simulink model "FullDynamics_Model2"  (R2018b)
settings: Solver=FixedStepAuto  StartTime=0.0  StopTime=inf  FixedStep=0.01  RelTol=1e-3
undefined symbols (not defined in the file): aMode
libraries: robotlib x6, autolibshared x1, autolibsharedcommon x1
settings Model: Creator=ivory  LastModifiedBy=ivory

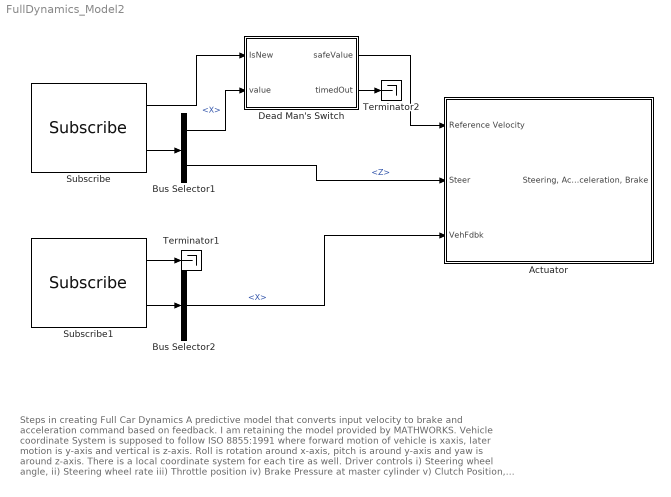
== system FullDynamics_Model2 ==
  note: Steps in creating Full Car Dynamics
      | A predictive model that converts input velocity
      | to brake and acceleration command based on feedback.
      | I am retaining the model provided by MATHWORKS.
      | Vehicle coordinate System is supposed to follow ISO
      | 8855:1991 where forward motion of vehicle is xaxis, later
      | motion is y-axis and vertical is z-axis. Roll is rotation around
      | x-axis, pitch is around y-axis and yaw is around z-axis. There
      | is a local coordinate system for each tire as well.
      | Driver controls i) Steering wheel angle, ii) Steering wheel rate
      | iii) Throttle position iv) Brake Pressure at master cylinder
      | v) Clutch Position, vi) Gear shift Position
      | Out of interests may be: i) Vehicle velocities ii) Vehicle Accelerations
      | iii) Vehicle angular velocities/rate iv) Steering wheel torque v) Engine
      | speed vi) Engine torque.
      | We need following main subcomponent: i) Chassis model ii) Tire model
      | iii) Suspension system iv) Steering system v) Driveline vi) Braking system
      | vii) Active Safety Systems
  Actuator : Subsystem
      mask Display: image('/home/ivory/Pictures/actuator.jpg');
  Bus Selector1 : BusSelector  OutputSignals=Linear.X,Angular.Z
  Bus Selector2 : BusSelector  OutputSignals=Linear.X
  Dead Man's Switch : Subsystem  TreatAsAtomicUnit=on  mask{stepSize=0.002, timeout=0.2}
      mask prompts: stepSize "Simulation step size"; timeout "Timeout (in seconds)"
      mask help: Interprets whether a new message has been recently received, and if so permits the data in 'value' to be passed through. Otherwise, 0 is outputted from 'safeValue'
      mask Help: Interprets whether a new message has been recently received, and if so permits the data in 'value' to be passed through. Otherwise, 0 is outputted from 'safeValue'
  Subscribe : robotlib/Subscribe  topicSource=Specify your own  topic=cmd_vel  messageType=geometry_msgs/Twist  sampleTime=-1  messageQueueLength=1
      settings: SourceProductBaseCode=RO
  Subscribe1 : robotlib/Subscribe  topicSource=Specify your own  topic=cmd_vel  messageType=geometry_msgs/Twist  sampleTime=-1  messageQueueLength=1
      settings: SourceProductBaseCode=RO
  Terminator1 : Terminator
  Terminator2 : Terminator
  wires:
  Bus Selector1/1 -> Dead Man's Switch/2(value)  "<X>"
  Subscribe/2 -> Bus Selector1/1
  Subscribe/1 -> Dead Man's Switch/1(IsNew)
  Dead Man's Switch/2(timedOut) -> Terminator2/1
  Dead Man's Switch/1(safeValue) -> Actuator/1(Reference Velocity)
  Bus Selector1/2 -> Actuator/2(Steer)  "<Z>"
  Subscribe1/2 -> Bus Selector2/1
  Subscribe1/1 -> Terminator1/1
  Bus Selector2/1 -> Actuator/3(VehFdbk)  "<X>"

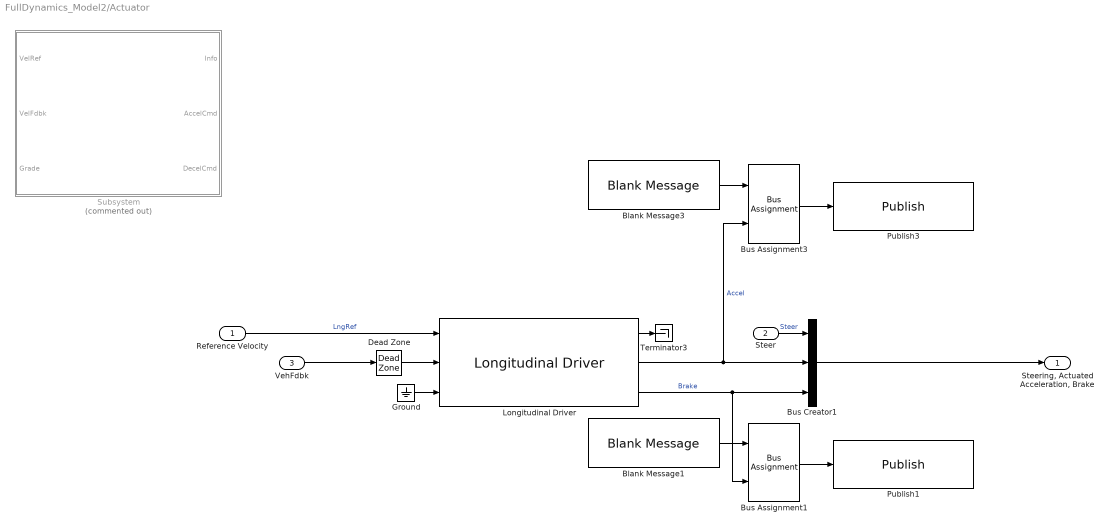
== system FullDynamics_Model2/Actuator ==
  Reference Velocity : Inport
  Steer : Inport  Port=2
  VehFdbk : Inport  Port=3
  Blank Message1 : robotlib/Blank Message  messageClass=Message  entityType=std_msgs/Float64  messageType=std_msgs/Float64  SampleTime=inf
      settings: SourceProductBaseCode=RO
  Blank Message3 : robotlib/Blank Message  messageClass=Message  entityType=std_msgs/Float64  messageType=std_msgs/Float64  SampleTime=inf
      settings: SourceProductBaseCode=RO
  Bus Assignment1 : BusAssignment  AssignedSignals=Data
  Bus Assignment3 : BusAssignment  AssignedSignals=Data
  Bus Creator1 : BusCreator  Inputs=3
  Dead Zone : DeadZone  LowerValue=-0.1  UpperValue=.1  SaturateOnIntegerOverflow=on
  Ground : Ground
  Longitudinal Driver : autolibshared/Longitudinal Driver  cntrlType=Predictive  shftType=None  velUnits=m/s  gearOut=off  Kp=5  Ki=5  Kff=.1  Kg=0  VehVelVec=[0 100]  KffVec=[.1 .1]  KpVec=[10 10]  KiVec=[5 5]  KgVec=[0 0]  m=1703.239  Kpt=3000  tau=.5  L=2  aR=200  bR=2.5  cR=.5  g=9.81  vnom=5  Kaw=1  tauerr=.075  tauPt=2  GearInit=0  tShift=.1  pdlVec=[0.1 0.4 0.5 0.9]  upShftTbl=[-1 12.9375 26.4375 39.9375 51.18749999999999 62.4375 72.84375 83.25;-1 16.3125 29.8125 43.3125 54.5624 65.8125 76.78125 87.75;-1 19.6875 33.1875 46.68749999999999 57.9375 69.1875 80.71875 92.25;-1 33 52.5 77.25 100.5 138.75 161.875 185]  dwnShftTbl=[1 9.5625 23.0625 36.5625 47.8125 59.0625 68.90625 78.75;1 12.9375 26.4375 39.9375 51.18749999999999 62.4375 72.84375 83.25;1 16.3125 29.8125 43.3125 54.562499 65.8125 76.78125 87.75;1 19.6875 33.1875 46.68749999999999 57.9375 69.1875 80.71875 92.25]  tClutch=.5  tRev=.5  tPark=120  aMode=2  UpGearVec="[0  1  2  3  4  5  6  7]"  DownGearVec="[1  2  3  4  5  6  7  8]"
      settings: SourceProductName=Powertrain Blockset  SourceProductBaseCode=PW
  Publish1 : robotlib/Publish  topicSource=Specify your own  topic=Brake_IN  messageType=std_msgs/Float64  messageQueueLength=1
      settings: SourceProductBaseCode=RO
  Publish3 : robotlib/Publish  topicSource=Specify your own  topic=Accel_IN  messageType=std_msgs/Float64  messageQueueLength=1
      settings: SourceProductBaseCode=RO
  Subsystem : Subsystem  Commented=on  mask(Longitudinal Driver){cntrlType=Predictive, shftType=None, gearOut=off, velUnits=m/s, Kp=10, Ki=5, Kff=0.1, Kg=0, VehVelVec=[0 100], KfVec=[.1 .1], KpVec=[10 10], KiVec=[5 5], KgVec=[0 0], m=1500, Kpt=10000, tau=0.2, L=4, aR=200, bR=2.5, cR=0.5, g=9.80665, vnom=5, Kaw=1, tauerr=0.01, tauPt=2, GearInit=0, tShift=0.1, pdlVec=[0.1 0.4 0.5 0.9], upShftTbl=[-1 12.9375 26.4375 39.9375 51.1875 62.4375 72.843 83.25; -1 16.3125 29.8125 43.3125 54.5624 65.8125 76.78125 87.75; -1 19.6875 33.1875 46.6875 57.9375 69.1875 80.71875 92.25; -1 33 52.5 77.25 100.5 138.75 161.875 185], dwnShftTbl=[ 1 9.5625 23.0625 36.5625 47.8125 59.0625 68.90625 78.75; 1 12.9375 26.4375 39.9375 51.1875 62.4375 72.84375 83.25; 1 16.3125 29.8125 43.3125 54.5625 65.8125 76.78125 87.75; 1 19.6875 33.1875 46.6875 57.9375 69.1875 80.71875 92.25], tClutch=0.5, tRev=0.5, tPark=120, aMode=aMode, UpGearVec=[0 1 2 3 4 5 6 7], DownGearVec=[1 2 3 4 5 6 7 8]}
      mask prompts: cntrlType "autoblks_shared:autoblkLongitudinalDriver:blkPrm_cntrlType"; shftType "autoblks_shared:autoblkLongitudinalDriver:blkPrm_shftType"; gearOut "autoblks_shared:autoblkLongitudinalDriver:blkPrm_gearOut"; velUnits "autoblks_shared:autoblkLongitudinalDriver:blkPrm_velUnits"; Kp "autoblks_shared:autoblkLongitudinalDriver:blkPrm_Kp"; Ki "autoblks_shared:autoblkLongitudinalDriver:blkPrm_Ki"; Kff "autoblks_shared:autoblkLongitudinalDriver:blkPrm_Kff"; Kg "autoblks_shared:autoblkLongitudinalDriver:blkPrm_Kg"; VehVelVec "autoblks_shared:autoblkLongitudinalDriver:blkPrm_VehVelVec"; KfVec "autoblks_shared:autoblkLongitudinalDriver:blkPrm_KfVec"; KpVec "autoblks_shared:autoblkLongitudinalDriver:blkPrm_KpVec"; KiVec "autoblks_shared:autoblkLongitudinalDriver:blkPrm_KiVec"; KgVec "autoblks_shared:autoblkLongitudinalDriver:blkPrm_KgVec"; m "autoblks_shared:autoblkLongitudinalDriver:blkPrm_m"; Kpt "autoblks_shared:autoblkLongitudinalDriver:blkPrm_Kpt"; tau "autoblks_shared:autoblkLongitudinalDriver:blkPrm_tau"; L "autoblks_shared:autoblkLongitudinalDriver:blkPrm_L"; aR "autoblks_shared:autoblkLongitudinalDriver:blkPrm_aR"; bR "autoblks_shared:autoblkLongitudinalDriver:blkPrm_bR"; cR "autoblks_shared:autoblkLongitudinalDriver:blkPrm_cR"; g "autoblks_shared:autoblkLongitudinalDriver:blkPrm_g"; vnom "autoblks_shared:autoblkLongitudinalDriver:blkPrm_vnom"; Kaw "autoblks_shared:autoblkLongitudinalDriver:blkPrm_Kaw"; tauerr "autoblks_shared:autoblkLongitudinalDriver:blkPrm_tauerr"; tauPt "autoblks_shared:autoblkLongitudinalDriver:blkPrm_tauPt"; GearInit "autoblks_shared:autoblkLongitudinalDriver:blkPrm_GearInit"; tShift "autoblks_shared:autoblkLongitudinalDriver:blkPrm_tShift"; pdlVec "autoblks_shared:autoblkLongitudinalDriver:blkPrm_pdlVec"; upShftTbl "autoblks_shared:autoblkLongitudinalDriver:blkPrm_upShftTbl"; dwnShftTbl "autoblks_shared:autoblkLongitudinalDriver:blkPrm_dwnShftTbl"; tClutch "autoblks_shared:autoblkLongitudinalDriver:blkPrm_tClutch"; tRev "autoblks_shared:autoblkLongitudinalDriver:blkPrm_tRev"; tPark "autoblks_shared:autoblkLongitudinalDriver:blkPrm_tPark"; UpGearVec "autoblks_shared:autoblkLongitudinalDriver:blkPrm_UpGearVec"; DownGearVec "autoblks_shared:autoblkLongitudinalDriver:blkPrm_DownGearVec"
      mask help: autoblks_shared:autoblkLongitudinalDriver:blkDesc
      mask init:
      | [~]=autosharedicon('autoliboperlong',gcb,0);
      mask Help: eval('autosharedhelp(''pbopmodlong'')');
      mask TypeOptions cntrlType: PI | Scheduled PI | Predictive
      mask TypeOptions shftType: None | Reverse, Neutral, Drive | Scheduled | External
      mask TypeOptions velUnits: VelRef/Unit
      mask DialogControl modeConfig Prompt: autoblks_shared:autoblkLongitudinalDriver:blkDlg_modeConfig
      mask DialogControl cntrlType Prompt: Control type, cntrlType:
      mask DialogControl shftType Prompt: Shift type, shftType:
      mask DialogControl gearOut Prompt: Output gear signal
      mask DialogControl velUnits Prompt: Reference and feedback units, velUnits :
      mask DialogControl CntrlParamPanel Prompt: autoblks_shared:autoblkLongitudinalDriver:blkDlg_CntrlParamPanel
      mask DialogControl PIParam Prompt: autoblks_shared:autoblkLongitudinalDriver:blkPrm_PIParam
      mask DialogControl Kp Prompt: Proportional gain, Kp []:
      mask DialogControl Ki Prompt: Integral gain, Ki []:
      mask DialogControl Kff Prompt: Velocity feed-forward, Kff []:
      mask DialogControl Kg Prompt: Grade feed-forward, Kg [1/deg]:
      mask DialogControl PISchedParam Prompt: autoblks_shared:autoblkLongitudinalDriver:blkPrm_PISchedParam
      mask DialogControl VehVelVec Prompt: Velocity gain breakpoints, VehVelVec:
      mask DialogControl KpVec Prompt: Proportional gain values, KpVec []:
      mask DialogControl KiVec Prompt: Integral gain values, KiVec []:
      mask DialogControl KgVec Prompt: Grade feed-forward values, KgVec [1/deg]:
      mask DialogControl PredParam Prompt: autoblks_shared:autoblkLongitudinalDriver:blkPrm_PredParam
      mask DialogControl m Prompt: Vehicle mass, m [kg]:
      mask DialogControl Kpt Prompt: Effective vehicle total tractive force, Kpt [N]:
      mask DialogControl tau Prompt: Driver response time, tau [s]:
      mask DialogControl L Prompt: Preview distance, L [m]:
      mask DialogControl aR Prompt: Rolling resistance coefficient, aR [N]:
      mask DialogControl bR Prompt: Rolling and driveline resistance coefficient, bR [N*s/m]:
      mask DialogControl cR Prompt: Aerodynamic drag coefficient, cR [N*s^2/m^2]:
      mask DialogControl g Prompt: Gravitational constant, g [m/s^2]:
      mask DialogControl vnom Prompt: Nominal speed, vnom [velUnits]:
      mask DialogControl Kaw Prompt: Anti-windup, Kaw []:
      mask DialogControl tauerr Prompt: Error filter time constant, tauerr [s]:
      mask DialogControl shiftParamPanel Prompt: autoblks_shared:autoblkLongitudinalDriver:blkDlg_shiftlParamPanel
      mask DialogControl GearInit Prompt: Initial gear, GearInit []:
      mask DialogControl tShift Prompt: Time required to shift, tShift [s]:
      mask DialogControl pdlVec Prompt: Up and down shift accelerator pedal positions, pdlVec []:
      mask DialogControl upShftTbl Prompt: Upshift velocity data table, upShftTbl [velUnits]:
      mask DialogControl dwnShftTbl Prompt: Downshift velocity data table, dwnShftTbl [velUnits]:
      mask DialogControl tClutch Prompt: Time required to shift, tClutch [s]:
      mask DialogControl tRev Prompt: Time required to engage reverse from neutral, tRev [s]:
      mask DialogControl tPark Prompt: Time required to engage park from neutral, tPark [s]:
      mask DialogControl UpGearVec Prompt: Upshift gear vector, UpGearVec []:
      mask DialogControl DownGearVec Prompt: Downshift gear vector, DownGearVec []:
      mask Display:
      | try
      |     IconInfo = autosharedicon('autoliboperlong', gcb, 4);
      | 
      |     image(IconInfo.image, IconInfo.position);
      | 
      |     for i = 1:numel(IconInfo.lconn)
      |         port_label('lconn', i, IconInfo.lconn{i})
      |     end
      | 
      |     for j = 1:numel(IconInfo.rconn)
      |         port_label('rconn', j, IconInfo.rconn{j})
      |     end
      | 
      |     for k = 1:numel(IconInfo.input)
      |         port_label('input', k, IconInfo.input{k})
      |     end
      | 
      |     for m = 1:numel(IconInfo.output)
      |         port_label('output', m, IconInfo.output{m})
      |     end
      | catch
      |     fprintf('Longitudinal \n Driver')
      | end
  Terminator3 : Terminator
  "Steering, Actuated Acceleration, Brake" : Outport
  wires:
  Longitudinal Driver/3 -> Bus Assignment1/2, Bus Creator1/3  "Brake"
  Ground/1 -> Longitudinal Driver/3
  Longitudinal Driver/1 -> Terminator3/1
  Dead Zone/1 -> Longitudinal Driver/2
  Bus Creator1/1 -> "Steering, Actuated Acceleration, Brake"/1
  Reference Velocity/1 -> Longitudinal Driver/1  "LngRef"
  Longitudinal Driver/2 -> Bus Assignment3/2, Bus Creator1/2  "Accel"
  Steer/1 -> Bus Creator1/1  "Steer"
  Blank Message3/1 -> Bus Assignment3/1
  Bus Assignment3/1 -> Publish3/1
  Bus Assignment1/1 -> Publish1/1
  Blank Message1/1 -> Bus Assignment1/1
  VehFdbk/1 -> Dead Zone/1

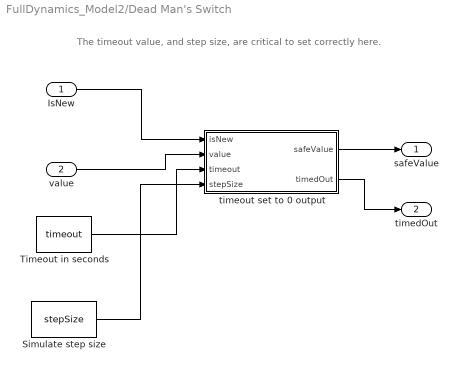
== system FullDynamics_Model2/Dead Man's Switch ==
  note: The timeout value, and step size, are critical to set correctly here.
  IsNew : Inport
  value : Inport  Port=2
  Simulate step size : Constant  Value=stepSize
  Timeout in seconds : Constant  Value=timeout
  timeout set to 0 output : MATLAB Function  TreatAsAtomicUnit=on
  safeValue : Outport  InitialOutput=[0]
  timedOut : Outport  Port=2  InitialOutput=[0]
  wires:
  IsNew/1 -> timeout set to 0 output/1(isNew)
  timeout set to 0 output/1(safeValue) -> safeValue/1
  value/1 -> timeout set to 0 output/2(value)
  Timeout in seconds/1 -> timeout set to 0 output/3(timeout)
  timeout set to 0 output/2(timedOut) -> timedOut/1
  Simulate step size/1 -> timeout set to 0 output/4(stepSize)

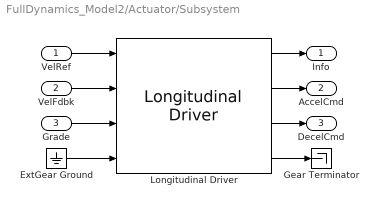
== system FullDynamics_Model2/Actuator/Subsystem ==
  VelRef : Inport  Unit=m/s
  VelFdbk : Inport  Port=2  Unit=m/s
  Grade : Inport  Port=3
  ExtGear Ground : Ground
  Gear Terminator : Terminator
  Longitudinal Driver : autolibsharedcommon/Longitudinal Driver  cntrlType=PI  shftType=None  vnom=vnom  Kp=Kp  Ki=Ki  Kaw=Kaw  Kff=Kff  Kg=Kg  tauerr=tauerr  tShift=tShift  tRev=tRev  tPark=tPark  pdlVec=pdlVec  upShftTbl=upShftTbl  dwnShftTbl=dwnShftTbl  GearInit=GearInit  tClutch=tClutch  VehVelVec=VehVelVec  KffVec=KffVec  KiVec=KiVec  KpVec=KpVec  KgVec=KgVec  m=m  Kpt=Kpt  Lvv=L  g=g  UpGearVec=UpGearVec  DownGearVec=DownGearVec  aMode=aMode  errUnit=m/s  aR=aR  bR=bR  cR=cR  tauPt=tauPt
      settings: SourceProductName=Powertrain Blockset  SourceProductBaseCode=PW
  Info : Outport  InitialOutput=0
  AccelCmd : Outport  Port=2
  DecelCmd : Outport  Port=3
  wires:
  Longitudinal Driver/4 -> Gear Terminator/1
  VelFdbk/1 -> Longitudinal Driver/2
  Grade/1 -> Longitudinal Driver/3
  ExtGear Ground/1 -> Longitudinal Driver/4
  Longitudinal Driver/1 -> Info/1
  Longitudinal Driver/3 -> DecelCmd/1
  VelRef/1 -> Longitudinal Driver/1
  Longitudinal Driver/2 -> AccelCmd/1

== matlab function FullDynamics_Model2/Dead Man's Switch/timeout set to 0 output ==
  data: isNew input; safeValue output; value input; timeout input; timedOut output; stepSize input
function [safeValue,timedOut] = fcn(isNew,value,timeout,stepSize)
%#codegen
persistent sinceLastMsg
timedOut=true;
if isempty(sinceLastMsg)
    sinceLastMsg=(timeout/stepSize)+1;
end

safeValue=0;
% if no new message
% after timeout, we output 0
if( isNew == true )
    sinceLastMsg = 0;
else
    sinceLastMsg = sinceLastMsg+1;
end

% Note: we require step size as an input here, and depend on our
% system being executed at a regular rate, or bad things will happen
if( sinceLastMsg < timeout/stepSize )
    timedOut = false;
end
    
if( timedOut == false )
    safeValue = value;
end
